simulink model "SimEstanque2a"  (R2020a)
settings: Solver=ode45  StartTime=0.0  StopTime=500  RelTol=1e-3
values from neighbouring files (symbols this model uses):
  tescalon = 100    [Prueba.m]
settings Model: Creator=rober  LastModifiedBy=maibe
settings SolverCC: ZeroCrossAlgorithm=Adaptive
settings DataIOCC: SaveFormat=StructureWithTime  ReturnWorkspaceOutputs=off
settings OptimizationCC: LifeSpan=inf
settings DebuggingCC: IgnoredZcDiagnostic=none  SFExecutionAtInitializationDiag=none  ArithmeticOperatorsInVariantConditions=warning
settings HardwareCC: ProdBitPerSizeT=32  ProdBitPerPtrDiffT=32  ProdWordSize=32  ProdHWDeviceType=Specified
settings SFSimCC: CustomCodeUndefinedFunction=UseInterfaceOnly
settings CodeAppCC: StateflowObjectComments=on

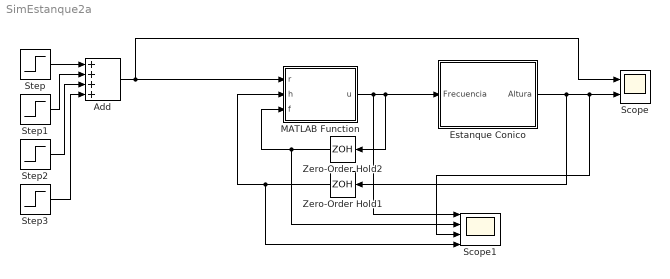
== system SimEstanque2a ==
  Add : Sum  Inputs=++++
  Estanque Conico : Subsystem
  MATLAB Function : MATLAB Function  TreatAsAtomicUnit=on
  Scope : Scope  NumInputPorts=2
  Scope1 : Scope  NumInputPorts=4
  Step : Step  Time=0  After=25  SampleTime=0
  Step1 : Step  Time=tescalon  After=10  SampleTime=0
  Step2 : Step  Time=2*tescalon  After=-5  SampleTime=0
  Step3 : Step  Time=3*tescalon  After=15  SampleTime=0
  Zero-Order Hold1 : ZeroOrderHold  SampleTime=10
  Zero-Order Hold2 : ZeroOrderHold  SampleTime=10
  wires:
  Step/1 -> Add/1
  Step1/1 -> Add/2
  Step2/1 -> Add/3
  Step3/1 -> Add/4
  Estanque Conico/1(Altura) -> Zero-Order Hold1/1, Scope1/3, Scope/2
  Add/1 -> MATLAB Function/1(r), Scope/1
  MATLAB Function/1(u) -> Estanque Conico/1(Frecuencia), Zero-Order Hold2/1, Scope1/1
  Zero-Order Hold2/1 -> Scope1/2, MATLAB Function/3(f)
  Zero-Order Hold1/1 -> Scope1/4, MATLAB Function/2(h)

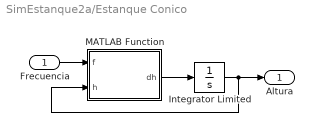
== system SimEstanque2a/Estanque Conico ==
  Frecuencia : Inport
  Integrator Limited : Integrator  InitialCondition=20  LimitOutput=on  LowerSaturationLimit=0
  MATLAB Function : MATLAB Function  TreatAsAtomicUnit=on
  Altura : Outport
  wires:
  Integrator Limited/1 -> MATLAB Function/2(h), Altura/1
  MATLAB Function/1(dh) -> Integrator Limited/1
  Frecuencia/1 -> MATLAB Function/1(f)

== matlab function SimEstanque2a/MATLAB Function ==
  data: r input; u output; h input; f input
function u = Controlador(r,h,f)

coder.extrinsic('ControladorOpt');
u=0;
u=ControladorOpt(r,h,f);
end

== matlab function SimEstanque2a/Estanque Conico/MATLAB Function ==
  data: f input; dh output; h input
function dh = fcn(f,h)
Fin=5.43*f+78.23;
Fout=20.21*sqrt(h);
Num=Fin-Fout;
Den=0.63*h^2+11.4*h+17.1;
dh = real(Num/Den);
